simulink model "p5p5cx"  (Simulink 8.9)
settings: Solver=ode45  StartTime=0.0  StopTime=5000  RelTol=1e-3  EnableMultiTasking=on
values from neighbouring files (symbols this model uses):
  K_pd = sqrt((0.01*T_f)^2+0.01)/K    [p5p5c.m]
  psi_ref = 30    [p5p5c.m]
  T_d = T    [p5p5c.m]
  T_f = -10/tan(130*pi/180)    [p5p5c.m]
libraries: simulink x2
settings Model: Creator=markh  LastModifiedBy=tikjetsa
settings DataIOCC: SignalLoggingName=sigsOut
settings OptimizationCC: InitFltsAndDblsToZero=on
settings DebuggingCC: SaveWithParameterizedLinksMsg=none  SignalResolutionControl=TryResolveAllWithWarning  MultiTaskDSMMsg=warning  MultiTaskCondExecSysMsg=none
settings HardwareCC: TargetBitPerPointer=64  TargetBitPerSizeT=64  TargetBitPerPtrDiffT=64  TargetLongLongMode=on  TargetIntDivRoundTo=Zero  TargetEndianess=LittleEndian  TargetWordSize=64  TargetHWDeviceType=MATLAB Host  ProdEqTarget=off
settings GRTTargetCC: TargetFcnLib=ansi_tfl_tmw.mat

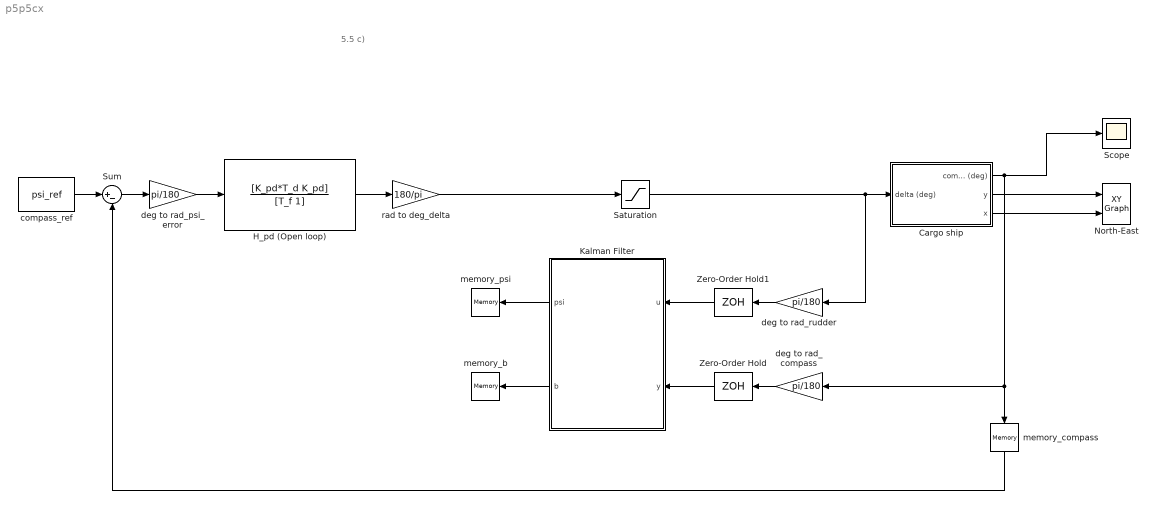
== system p5p5cx ==
  note: 5.5 c)
  Cargo ship : Subsystem  mask(Simple shipmodel for a cargo ship){noise=on, current=off, logic=on}
      mask prompts: noise "measurement noise"; logic "waves"
      mask help:
      | Measurement noise:
      | 	checked = noise on
      | 	unchecked = noise off
      |
      | Current:
      | 	checked = current on
      | 	unchecked = current off
      |
      | Waves:
      | 	checked = waves on
      | 	unchecked = waves off
      |
      | Author: Jørgen Spjøtvold, 9/10-2003
      | TTK 4115 Linear system theory.
      | Modified by Jostein Bakkeheim 26/10-2006
  H_pd (Open loop) : TransferFcn  Numerator=[K_pd*T_d K_pd]  Denominator=[T_f 1]
  Kalman Filter : MATLAB Function  TreatAsAtomicUnit=on
  North-East : simulink/Sinks/XY Graph  xmin=-5000  xmax=5000  ymin=-5000  ymax=5000  st=-1
  Saturation : Saturate  UpperLimit=45  LowerLimit=-45
  Scope : Scope
  Sum : Sum  Inputs=|+-
  Zero-Order Hold : ZeroOrderHold  SampleTime=0.1
  Zero-Order Hold1 : ZeroOrderHold  SampleTime=0.1
  compass_ref : Constant  Value=psi_ref
  deg to rad_compass : Gain  Gain=pi/180
  deg to rad_psi_error : Gain  Gain=pi/180
  deg to rad_rudder : Gain  Gain=pi/180
  memory_b : Memory
  memory_compass : Memory
  memory_psi : Memory
  rad to deg_delta : Gain  Gain=180/pi
  wires:
  Cargo ship/3(x) -> North-East/2
  Cargo ship/2(y) -> North-East/1
  H_pd (Open loop)/1 -> rad to deg_delta/1
  deg to rad_psi_error/1 -> H_pd (Open loop)/1
  Cargo ship/1(compass (deg)) -> deg to rad_compass/1, memory_compass/1, Scope/1
  Sum/1 -> deg to rad_psi_error/1
  compass_ref/1 -> Sum/1
  Saturation/1 -> Cargo ship/1(delta (deg)), deg to rad_rudder/1
  Zero-Order Hold/1 -> Kalman Filter/2(y)
  Zero-Order Hold1/1 -> Kalman Filter/1(u)
  rad to deg_delta/1 -> Saturation/1
  Kalman Filter/1(psi) -> memory_psi/1
  Kalman Filter/2(b) -> memory_b/1
  memory_compass/1 -> Sum/2
  deg to rad_rudder/1 -> Zero-Order Hold1/1
  deg to rad_compass/1 -> Zero-Order Hold/1

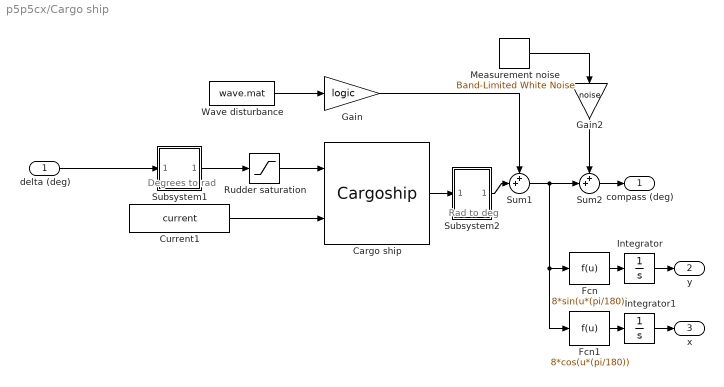
== system p5p5cx/Cargo ship ==
  note: Degrees to rad
  note: Rad to deg
  delta (deg) : Inport
  Cargo ship : S-Function  FunctionName=Cargoship  SFunctionDeploymentMode=off  EnableBusSupport=off  mask(Cargo ship){}
      mask help:
      | S-function which simulates a cargo ship.
      |
      | Author: Jørgen Spjøtvold
      | 20.10-2003
      | Modified by Jostein Bakkeheim 27.10.2006
  Current1 : Constant  Value=current
  Fcn : Fcn  Expr=8*sin(u*(pi/180))
  Fcn1 : Fcn  Expr=8*cos(u*(pi/180))
  Gain : Gain  Gain=logic  SaturateOnIntegerOverflow=on  OutDataTypeStr=Inherit: Same as input  ParamDataTypeStr=Inherit: Same as input
  Gain2 : Gain  Gain=noise  SaturateOnIntegerOverflow=on  OutDataTypeStr=Inherit: Same as input  ParamDataTypeStr=Inherit: Same as input
  Integrator : Integrator
  Integrator1 : Integrator
  Measurement noise : simulink/Sources/Band-Limited White Noise  Cov=[0.001]  Ts=.5  seed=[23341]
  Rudder saturation : Saturate  UpperLimit=45*(pi/180)  LowerLimit=-45*(pi/180)
  Subsystem1 : Subsystem  mask(degrees to radians){}
      mask help: Converts degrees to radians
      mask Display: fprintf('D2R');
  Subsystem2 : Subsystem  mask(radians to degrees){}
      mask help: Converts radians to degrees
      mask Display: fprintf('R2D');
  Sum1 : Sum  Inputs=++|  SaturateOnIntegerOverflow=on
  Sum2 : Sum  Inputs=++|  SaturateOnIntegerOverflow=on
  Wave disturbance : FromFile  FileName=wave.mat  SampleTime=0
  compass (deg) : Outport
  y : Outport  Port=2
  x : Outport  Port=3
  wires:
  delta (deg)/1 -> Subsystem1/1(In1)
  Fcn/1 -> Integrator/1
  Integrator/1 -> y/1
  Fcn1/1 -> Integrator1/1
  Integrator1/1 -> x/1
  Wave disturbance/1 -> Gain/1
  Subsystem2/1(Out1) -> Sum1/2
  Gain/1 -> Sum1/1
  Sum1/1 -> Fcn/1, Fcn1/1, Sum2/2
  Cargo ship/1 -> Subsystem2/1(In1)
  Subsystem1/1(Out1) -> Rudder saturation/1
  Rudder saturation/1 -> Cargo ship/1
  Sum2/1 -> compass (deg)/1
  Measurement noise/1 -> Gain2/1
  Gain2/1 -> Sum2/1
  Current1/1 -> Cargo ship/2

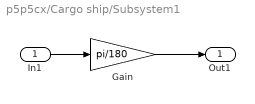
== system p5p5cx/Cargo ship/Subsystem1 ==
  In1 : Inport
  Gain : Gain  Gain=pi/180  SaturateOnIntegerOverflow=on  OutDataTypeStr=Inherit: Same as input  ParamDataTypeStr=Inherit: Same as input
  Out1 : Outport
  wires:
  Gain/1 -> Out1/1
  In1/1 -> Gain/1

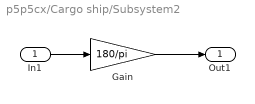
== system p5p5cx/Cargo ship/Subsystem2 ==
  In1 : Inport
  Gain : Gain  Gain=180/pi  SaturateOnIntegerOverflow=on  OutDataTypeStr=Inherit: Same as input  ParamDataTypeStr=Inherit: Same as input
  Out1 : Outport
  wires:
  Gain/1 -> Out1/1
  In1/1 -> Gain/1

== matlab function Kalman Filter ==
  data: u input double; psi output double; y input double; b output double; data parameter double
function [psi,b]=kalman_matl_func(u,y,data)
%coder.extrinsic('evalin')
persistent init_flag A_k B_k C_k E_k I_k P_pri Q_k R_k x_pri;

if isempty(init_flag)
    init_flag=1;
    %data=evalin('base', 'data');
    %evalin('base',[[A_k, B_k, C_k, E_k, I_k, P_pri, Q_k, R_k, x_pri] ' = ' deal(data.A_d,data.B_d,data.C_d, data.E_d, data.I, data.P_0, data.Q, data.R_rad_d, data.x_0) ';'])
    [A_k, B_k, C_k, E_k, I_k, P_pri, Q_k, R_k, x_pri] = deal(data.A_d ,data.B_d, data.C_d, data.E_d, data.I, data.P_0, data.Q, data.R_rad_d, data.x_0);
    %[A_k, B_k, C_k, E_k, I_k, P_pri, Q_k, R_k, x_pri] = deal(A_d,B_d,C_d, E_d, I, P_0, Q, R_rad_d, x_0);
    
end
% 1:Compute Kalman Gain
L_k=P_pri*C_k'*inv(C_k*P_pri*C_k' + R_k);

% 2: Update estimate with measurement
x_post=x_pri+L_k*(y-C_k*x_pri);

% 3 - Update error covariance matrix
P_post = (I_k - L_k*C_k)*P_pri*(I_k - L_k*C_k)'+L_k*R_k*L_k';

% 4 - Project ahead
x_pri = A_k*x_post + B_k*u;
P_pri = A_k*P_post*A_k' + E_k*Q_k*E_k';

% Output
psi = x_post(3); b = x_post(5);

end
